simulink model "PD_Control"  (R2021b)
settings: Solver=VariableStepAuto  StartTime=0.0  StopTime=10  RelTol=1e-3
undefined symbols (not defined in the file or in its folder): Kp, q_dq_init, qd
settings Model: Creator=Yafei Ou  LastModifiedBy=ouyaf

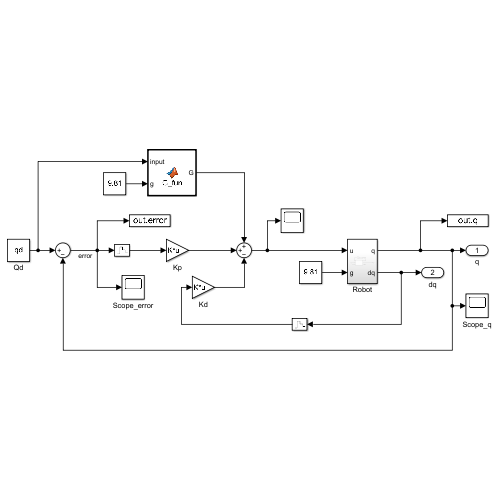
[thumbnail: Simulink's stored preview of the top-level diagram]
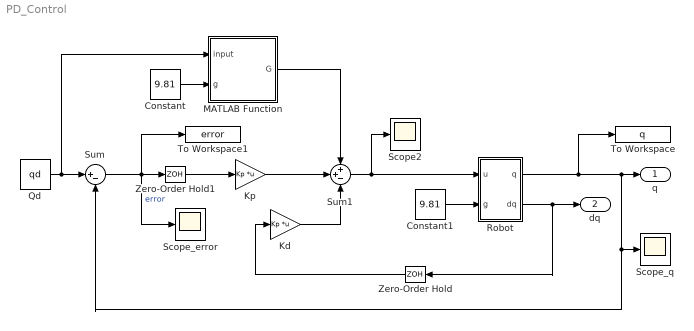
== system PD_Control ==
  Constant : Constant  Value=9.81
  Constant1 : Constant  Value=9.81
  Kd : Gain  Gain=Kp  Multiplication=Matrix(K*u)
  Kp : Gain  Gain=Kp  Multiplication=Matrix(K*u)
  MATLAB Function : MATLAB Function  TreatAsAtomicUnit=on
  Qd : Constant  Value=qd
  Robot : Subsystem
  Scope2 : Scope
  Scope_error : Scope
  Scope_q : Scope
  Sum : Sum  Inputs=|+-
  Sum1 : Sum  Inputs=++-
  To Workspace : ToWorkspace  VariableName=q  SaveFormat=Timeseries  SampleTime=-1
  To Workspace1 : ToWorkspace  VariableName=error  SaveFormat=Timeseries  SampleTime=-1
  Zero-Order Hold : ZeroOrderHold  SampleTime=0.01
  Zero-Order Hold1 : ZeroOrderHold  SampleTime=0.01
  q : Outport
  dq : Outport  Port=2
  wires:
  Qd/1 -> MATLAB Function/1(input), Sum/1
  Kd/1 -> Sum1/3
  Kp/1 -> Sum1/2
  MATLAB Function/1(G) -> Sum1/1
  Sum1/1 -> Scope2/1, Robot/1(u)
  Constant/1 -> MATLAB Function/2(g)
  Sum/1 -> To Workspace1/1, Zero-Order Hold1/1, Scope_error/1  "error"
  Robot/2(dq) -> Zero-Order Hold/1, dq/1
  Constant1/1 -> Robot/2(g)
  Zero-Order Hold/1 -> Kd/1
  Robot/1(q) -> To Workspace/1, q/1, Sum/2, Scope_q/1
  Zero-Order Hold1/1 -> Kp/1

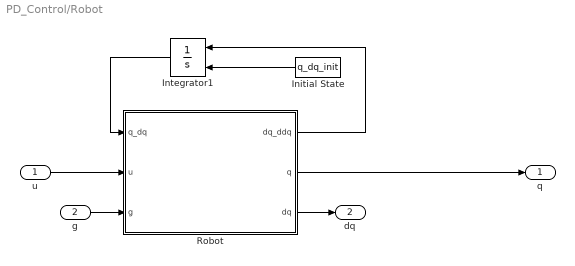
== system PD_Control/Robot ==
  u : Inport
  g : Inport  Port=2
  Initial State : Constant  Value=q_dq_init
  Integrator1 : Integrator  InitialConditionSource=external
  Robot : MATLAB Function  TreatAsAtomicUnit=on
  q : Outport
  dq : Outport  Port=2
  wires:
  u/1 -> Robot/2(u)
  Integrator1/1 -> Robot/1(q_dq)
  Robot/1(dq_ddq) -> Integrator1/1
  Robot/2(q) -> q/1
  Robot/3(dq) -> dq/1
  Initial State/1 -> Integrator1/2
  g/1 -> Robot/3(g)

== matlab function PD_Control/MATLAB Function ==
  data: input input; G output; g input
function G = G_fun(input,g)
%G_FUN
%    G = G_FUN(Q1,Q2,Q3,Q4,Q5,Q6,G)

%    This function was generated by the Symbolic Math Toolbox version 8.7.
%    16-Mar-2022 16:42:47

q1 = input(1);
q2 = input(2);
q3 = input(3);
q4 = input(4);
q5 = input(5);
q6 = input(6);


t2 = cos(q1);
t3 = cos(q2);
t4 = cos(q4);
t5 = cos(q5);
t6 = cos(q6);
t7 = sin(q1);
t8 = sin(q2);
t9 = sin(q4);
t10 = sin(q5);
t11 = sin(q6);
mt1 = [g.*t2.*(1.07e+2./1.0e+3)-g.*t7.*(3.0./5.0e+1)+g.*t3.*t7.*5.13502e-1+g.*t7.*t8.*1.895e-1+g.*q3.*t3.*t7.*(1.9e+1./5.0e+1)+g.*t3.*t5.*t7.*1.91e-4+(g.*t2.*t4.*t11)./1.0e+4-g.*t2.*t9.*t10.*1.91e-4+(g.*t3.*t5.*t6.*t7)./1.0e+4-(g.*t2.*t6.*t9.*t10)./1.0e+4-g.*t4.*t7.*t8.*t10.*1.91e-4-(g.*t7.*t8.*t9.*t11)./1.0e+4-(g.*t4.*t6.*t7.*t8.*t10)./1.0e+4];
mt2 = [g.*t2.*t3.*(-1.895e-1)+g.*t2.*t8.*5.13502e-1+g.*q3.*t2.*t8.*(1.9e+1./5.0e+1)+g.*t2.*t5.*t8.*1.91e-4+g.*t2.*t3.*t4.*t10.*1.91e-4+(g.*t2.*t5.*t6.*t8)./1.0e+4+(g.*t2.*t3.*t9.*t11)./1.0e+4+(g.*t2.*t3.*t4.*t6.*t10)./1.0e+4;g.*t2.*t3.*(-1.9e+1./5.0e+1)];
mt3 = [g.*t4.*t7.*t10.*(-1.91e-4)-(g.*t7.*t9.*t11)./1.0e+4+(g.*t2.*t4.*t8.*t11)./1.0e+4-(g.*t4.*t6.*t7.*t10)./1.0e+4-g.*t2.*t8.*t9.*t10.*1.91e-4-(g.*t2.*t6.*t8.*t9.*t10)./1.0e+4;g.*t2.*t3.*t10.*1.91e-4-g.*t5.*t7.*t9.*1.91e-4+g.*t2.*t4.*t5.*t8.*1.91e-4+(g.*t2.*t3.*t6.*t10)./1.0e+4-(g.*t5.*t6.*t7.*t9)./1.0e+4+(g.*t2.*t4.*t5.*t6.*t8)./1.0e+4];
mt4 = [(g.*t4.*t6.*t7)./1.0e+4+(g.*t2.*t3.*t5.*t11)./1.0e+4+(g.*t2.*t6.*t8.*t9)./1.0e+4+(g.*t7.*t9.*t10.*t11)./1.0e+4-(g.*t2.*t4.*t8.*t10.*t11)./1.0e+4];
G = [mt1;mt2;mt3;mt4];

== matlab function PD_Control/Robot/Robot ==
  data: q_dq input; dq_ddq output; u input; q output; dq output; g input
function [dq_ddq,q,dq] = fcn(q_dq,u,g)
    q = q_dq(1:length(q_dq)/2);
    dq = q_dq(length(q_dq)/2+1:length(q_dq));
    g_num = g;

%     in1 = q;
%     in2 = [q;dq];
%     in3 = [q;g_num];
%     in1 = mat2cell(in1,ones(numel(in1),1),1);
%     in2 = mat2cell(in2,ones(numel(in2),1),1);
%     in3 = mat2cell(in3,ones(numel(in3),1),1);


    M = M_fun(q);
    C = C_fun(q,dq);
    G = G_fun(q,g_num);

    ddq = M\(u - C - G);
    
    dq_ddq = [dq;ddq];

end
